simulink model "test_ppm_rc_input_02"  (Simulink 8.8)
settings: Solver=FixedStepDiscrete  StartTime=0.0  StopTime=10.0  FixedStep=0.3  RelTol=1e-3  EnableMultiTasking=on
InitFcn:
  | px4_ap1_mdl_callback('check_model');
libraries: px4_ap1_px4setup_lib x1, px4_ap1_rc_ppm_input_lib x1
settings Model: Creator=Privat  LastModifiedBy=Privat
settings OptimizationCC: ExpressionDepthLimit=2147483647  InitFltsAndDblsToZero=on  LifeSpan=1
settings DebuggingCC: SolverPrmCheckMsg=warning  InheritedTsInSrcMsg=none  StrictBusMsg=Warning
settings RTWCC: SystemTargetFile=px4_ap1.tlc  GenCodeOnly=on  GenerateMakefile=off
settings CodeAppCC: IgnoreCustomStorageClasses=off  CustomSymbolStrType=$N$R$M  InternalIdentifier=Classic
settings STFCustomTargetCC: ModelReferenceCompliant=off  IncludeMdlTerminateFcn=off  CombineOutputUpdateFcns=on  ERTCustomFileBanners=on  SupportContinuousTime=off  SupportNonInlinedSFcns=off  RemoveResetFunc=on  MATLABClassNameForMDSCustomization=Simulink.SoftwareTarget.ERTCustomization  CPPClassGenCompliant=on  GRTInterface=off  SystemTargetFile=px4_ap1.tlc
settings ERTTargetCC: MultiwordLength=2048  ModelReferenceCompliant=off  ParMdlRefBuildCompliant=off  CompOptLevelCompliant=off  ConcurrentExecutionCompliant=off  IncludeMdlTerminateFcn=off  ERTFirstTimeCompliant=off  ModelStepFunctionPrototypeControlCompliant=off  UseToolchainInfoCompliant=off  ERTSrcFileBannerTemplate=px4_ap1_code_template.cgt  ERTHdrFileBannerTemplate=px4_ap1_code_template.cgt  ERTDataSrcFileTemplate=px4_ap1_code_template.cgt  ERTDataHdrFileTemplate=px4_ap1_code_template.cgt  ERTCustomFileTemplate=px4_ap1_main.tlc  ConvertIfToSwitch=off  SuppressUnreachableDefaultCases=off

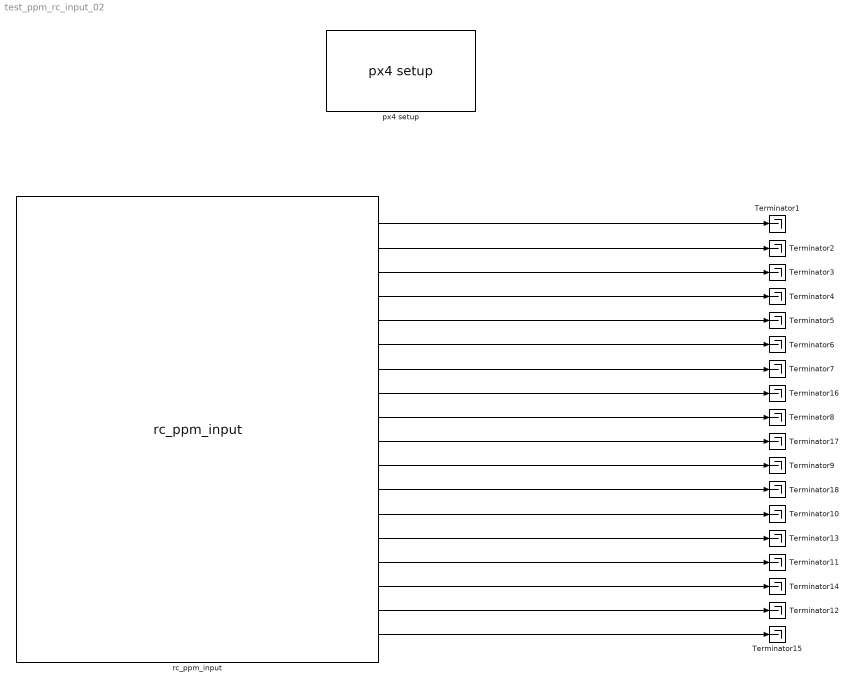
== system test_ppm_rc_input_02 ==
  Terminator{1..18} (18 alike) : Terminator
  px4 setup : px4_ap1_px4setup_lib/px4 setup  SampleTimeValue=0.3  cbBuild=on  cbUpload=off  cbPort=COM0  cpuLoad=on  debugmode=on
  rc_ppm_input : px4_ap1_rc_ppm_input_lib/rc_ppm_input  Description=Setup for PX4 native software  ch1=on  ch2=on  ch3=on  ch4=on  ch5=on  ch6=on  ch7=on  ch8=on  ch9=on  ch10=on  ch11=on  ch12=on  ch13=on  ch14=on  ch15=on  ch16=on  ch17=on  ch18=on
  wires:
  rc_ppm_input/1 -> Terminator1/1
  rc_ppm_input/18 -> Terminator15/1
  rc_ppm_input/2 -> Terminator2/1
  rc_ppm_input/3 -> Terminator3/1
  rc_ppm_input/4 -> Terminator4/1
  rc_ppm_input/5 -> Terminator5/1
  rc_ppm_input/6 -> Terminator6/1
  rc_ppm_input/7 -> Terminator7/1
  rc_ppm_input/8 -> Terminator16/1
  rc_ppm_input/9 -> Terminator8/1
  rc_ppm_input/10 -> Terminator17/1
  rc_ppm_input/11 -> Terminator9/1
  rc_ppm_input/12 -> Terminator18/1
  rc_ppm_input/13 -> Terminator10/1
  rc_ppm_input/14 -> Terminator13/1
  rc_ppm_input/15 -> Terminator11/1
  rc_ppm_input/16 -> Terminator14/1
  rc_ppm_input/17 -> Terminator12/1
